simulink model "bidirection_buck_boost"  (R2025a)
settings: Solver=VariableStepAuto  StartTime=0.0  StopTime=0.1  MaxStep=1e-7  RelTol=1e-3
libraries: ee_lib x12, nesl_utility x12, fl_lib x11, spsPWMGeneratorDCDCLib x4, spsPVArrayLib x1, spspowerguiLib x1
settings Model: Creator=GNKRISHNAN  LastModifiedBy=GNKRISHNAN

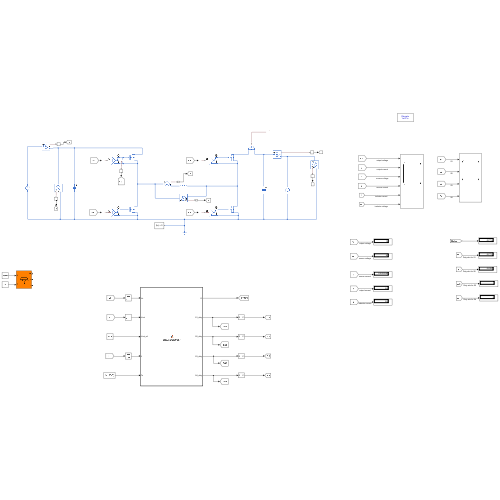
[thumbnail: Simulink's stored preview of the top-level diagram]
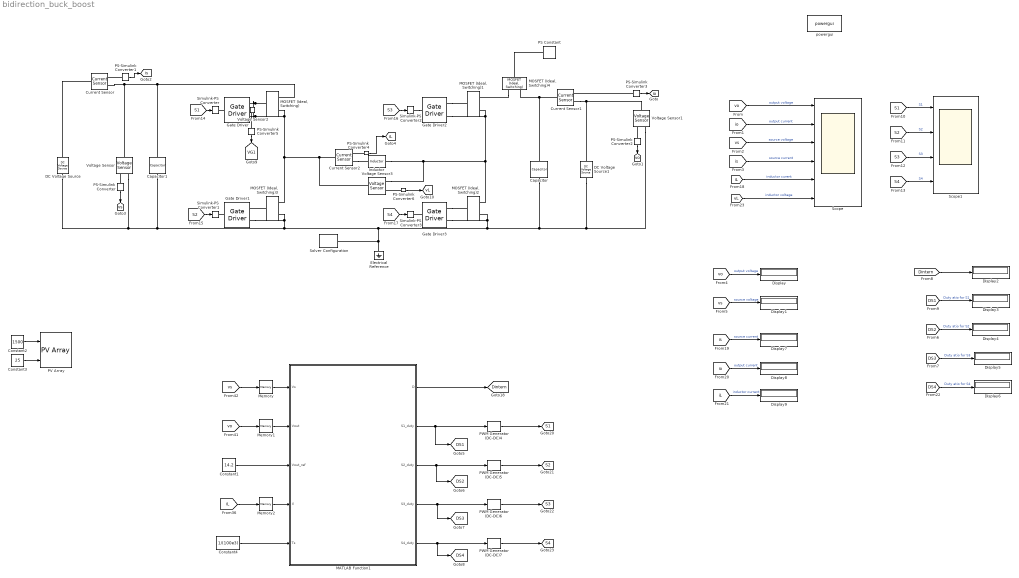
== system bidirection_buck_boost ==
  Capacitor : fl_lib/Electrical/Electrical Elements/Capacitor  c=120e-6 F  r=1e-6 Ohm  g=0 1/Ohm  i_specify=off  i_priority=None  i=0 A  i_nominal_specify=off  i_nominal_value=1  i_nominal_unit=A  v_specify=off  v_priority=None  v=0 V  v_nominal_specify=off  v_nominal_value=1  v_nominal_unit=V  vc_specify=on  vc_priority=High  vc=12 V  vc_nominal_specify=off  vc_nominal_value=1  vc_nominal_unit=V
  Capacitor1 : fl_lib/Electrical/Electrical Elements/Capacitor  c=400e-6 F  r=1e-6 Ohm  g=0 1/Ohm  i_specify=off  i_priority=None  i=0 A  i_nominal_specify=off  i_nominal_value=1  i_nominal_unit=A  v_specify=off  v_priority=None  v=0 V  v_nominal_specify=off  v_nominal_value=1  v_nominal_unit=V  vc_specify=off  vc_priority=High  vc=0 V  vc_nominal_specify=off  vc_nominal_value=1  vc_nominal_unit=V
  Constant1 : Constant  Value=14.2
  Constant2 : Constant  Value=1500
  Constant3 : Constant  Value=25
  Constant4 : Constant  Value=1/(100e3)
  Current Sensor : fl_lib/Electrical/Electrical Sensors/Current Sensor
  Current Sensor1 : fl_lib/Electrical/Electrical Sensors/Current Sensor
  Current Sensor2 : fl_lib/Electrical/Electrical Sensors/Current Sensor
  DC Voltage Source : ee_lib/Additional Components/SPICE Sources/DC Voltage Source  DC=20 V
  DC Voltage Source1 : ee_lib/Additional Components/SPICE Sources/DC Voltage Source  DC=12 V
  Display{,1..9} (10 alike) : Display
  Electrical Reference : fl_lib/Electrical/Electrical Elements/Electrical Reference
  Gate Driver{,1..3} (4 alike) : ee_lib/Semiconductors & Converters/Gate Driver  port_option=ee.enum.controlport.ps  uHigh=2.0 V  uLow=0.8 V  uHighValue=0.7  uLowValue=0.3  vHigh=15 V  vLow=0 V  tHigh=300 ns  tLow=300 ns  parameterization=ee.enum.semiconductors.gateDriverParam.outputImpedance  rHigh=2 Ohm  rLow=2 Ohm  tRise=20 ns  tFall=20 ns  cLoad=10 nF  ZonTime_specify=off  ZonTime_priority=None  ZonTime=0 s  ZoffTime_specify=off  ZoffTime_priority=None  ZoffTime=0 s
      settings: InternalSimscapePortConfiguration="{\"Bottom\":[],\"Left\":[{\"id\":\"u\",\"label\":\"u\",\"type\":\"input\"}],\"Right\":[{\"id\":\"G\",\"label\":\"G\",\"type\":\"foundation.electrical.electrical\"},{\"id\":\"S\",\"label\":\"S\",\"type\":\"foundation.electrical.electrical\"}],\"Top\":[]}"
  Inductor : ee_lib/Passive/Inductor  l=110e-6 H  enable_L_tol=ee.enum.toleranceApplication.none  L_tol=20  tol_distribution=ee.enum.toleranceDistribution.uniform  nSigma=4  r=0 Ohm  g=1e-9 1/Ohm  enable_operating_limits=ee.enum.enable.no  operating_limit_action=ee.enum.passive.reportOpLim.warn  max_working_current=1 A  power_rating=1 W  i_L_specify=off  i_L_priority=High  i_L=0 A  i_L_nominal_specify=off  i_L_nominal_value=1  i_L_nominal_unit=A
  MATLAB Function1 : MATLAB Function  TreatAsAtomicUnit=on  SystemSampleTime=1/(100e3)
  MOSFET (Ideal, Switching){,1..3} (4 alike) : ee_lib/Semiconductors & Converters/MOSFET (Ideal, Switching)  port_option=ee.enum.controlport.elec  Rds=0.01 Ohm  Goff=1e-6 1/Ohm  Vth=2 V  diode_param=ee.enum.semiconductors.protectionDiode.nodynamics  diode_Vf=0.8 V  diode_Ron=0.001 Ohm  diode_Goff=1e-5 1/Ohm  diode_C=50e-9 F  diode_iRM=-235 A  diode_iF=300 A  diode_idot=-50 A/us  diode_trr_param=ee.enum.converters.diodeReverseParam.trr_factor  diode_trr_factor=3  diode_trr=15 us  diode_Qrr=1500 s*uA  ids_specify=off  ids_priority=None  ids=0 A  ids_nominal_specify=off  ids_nominal_value=1  ids_nominal_unit=A  vds_specify=off  vds_priority=None  vds=0 V  vds_nominal_specify=off  vds_nominal_value=1  vds_nominal_unit=V  vgs_specify=off  vgs_priority=None  vgs=0 V  vgs_nominal_specify=off  vgs_nominal_value=1  vgs_nominal_unit=V  thermal_loss_option=ee.enum.converters.thermalLossOption.constantvalues  Von_data=[0, 1.8, 3.2, 6, 10, 16; 0, 2, 5.5, 9.5, 15, 25] V  Tj=[298.15, 448.15] K  Iout_data=[0, 20, 40, 60, 80, 100] A  Eon_data=[0, 55.04, 124.57, 235.53, 362.12; 0, 71.25, 161.25, 304.88, 468.75] * 1e-6 J  Eoff_data=[0, 18, 30, 56.1, 76.5; 0, 22.5, 37.5, 70.13, 95.63] * 1e-6 J  Eon_data_3D=[zeros(2, 5, 3)] J  Eoff_data_3D=[zeros(2, 5, 3)] J  Tj_loss=[298.15, 448.15] K  Iout_data_loss=[0, 10, 20, 30, 40] A  tabulateWithVds=false  Vds_loss=[0, 150, 300] V  Eon_scalar=22.86e-3 J  Eoff_scalar=17.14e-3 J  Voff=300 V  Iout_scalar=600 A  useCurrentFromPreviousCycle=false  useVoltageFromPreviousCycle=false  diodeModelType=ee.enum.converters.diodeModelType.pwl  diodeTableType=ee.enum.diode.tableType.IfMat  diode_ReverseIVType=ee.enum.diode.diodeReverseIV.constant  diode_IfMat=[.07, .12, .19, 1.75, 4.24, 7.32, 11.2; .16, .3, .72, 2.14, 4.02, 6.35, 9.12] A  diode_VfMat=[.9, 1.15, 1.25, 1.5, 1.75, 2.17, 2.6, 2.85; .58, .68, .75, 1.1, 1.38, 1.77, 2.27, 2.7] V  diode_TjVec=[25, 125] degC  diode_VfVec=[.5, .7, .9, 1.3, 1.7, 2.1, 2.5] V  diode_IfVec=[.1, .2, .5, 1, 2, 4, 7, 10] A  diode_IrMat=[1e-06, 2e-06, 5e-06, 1e-05, 2.5e-05, 5e-05, .0001; 2e-06, 5e-06, 1e-05, 4e-05, 8e-05, .0002, .0005] A  diode_VrMat=[10, 100, 200, 250, 300, 325, 350; 10, 70, 160, 220, 270, 300, 320] V  diode_VrVec=[10, 20, 40, 50, 70, 80, 100] V  diode_IrVec=[1e-06, 2e-06, 5e-06, 1e-05, 2e-05, 5e-05, .0001] A  diode_Vr=-600 V  diode_Ls=150 nH  diode_Erec=0.03 J  diode_rec_loss_model=ee.enum.diode.reverseRecoveryModel.fixed  diode_ErecVal=0 J  diode_scaleWithIandV=true  diode_ErecMat=zeros(2, 3) J  diode_TjrecVec=[298.15, 398.15] K  diode_IfrecVec=[.1, 1, 10] A  diode_IrecVal=10 A  diode_VrecVal=10 V  diode_tFilter=1 / 1000 / 100 s  separateThermalPortForDiode=false  thermal_network_parameterization=ee.enum.thermalNetworkTopology.external  Rth=[.03, .2] K/W  Rth_Cauer=[.03, .1, .2] K/W  Rth_Foster=[.08, .14, .22, .16] K/W  thermal_mass_parameterization=ee.enum.thermalNetwork.timeconstant  thermal_mass=[3, 25] J/K  thermal_mass_Cauer=[3, 10, 25] J/K  thermal_mass_Foster=[.001, .005, .05, .5] J/K  thermal_time_constant=[.1, 5] s  thermal_time_constant_Cauer=[.1, 1, 5] s  thermal_time_constant_Foster=[7e-05, .0007, .01, .08] s  thermal_mass_initial_temperatures=[25, 25] degC  thermal_mass_initial_temperatures_Cauer=[25, 25, 25] degC  junction_thermal_mass=0.1 J/K  Tvec_initial_Foster=[25, 25, 25, 25] degC  RthDiode=[.03, .2] K/W  RthCauerDiode=[.03, .1, .2] K/W  RthFosterDiode=[.03, .2] K/W  thermalMassDiode=[3, 25] J/K  thermalMassCauerDiode=[3, 10, 25] J/K  thermalMassFosterDiode=[33, 50] J/K  thermalTauDiode=[.1, 5] s  thermalTauCauerDiode=[.1, 1, 5] s  thermalTauFosterDiode=[1, 10] s  thermalMassInitTempDiode=[25, 25] degC  thermalMassInitTempCauerDiode=[25, 25, 25] degC  junctionthermalMassDiode=0.1 J/K  TVecInitialFosterDiode=[25, 25, 25, 25] degC  no_thermal_network=0  mosfet_junction_temperature_specify=off  mosfet_junction_temperature_priority=None  mosfet_junction_temperature=25 degC  mosfet_junction_temperature_nominal_specify=off  mosfet_junction_temperature_nominal_value=1  mosfet_junction_temperature_nominal_unit=degC  diode_junction_temperature_specify=off  diode_junction_temperature_priority=None  diode_junction_temperature=25 degC  diode_junction_temperature_nominal_specify=off  diode_junction_temperature_nominal_value=1  diode_junction_temperature_nominal_unit=degC  Qj_specify=off  Qj_priority=None  Qj=0 W  Qj_nominal_specify=off  Qj_nominal_value=1  Qj_nominal_unit=W  accumulatedSwitchingLosses_specify=off  accumulatedSwitchingLosses_priority=None  accumulatedSwitchingLosses=0 J
      settings: InternalSimscapePortConfiguration="{\"Bottom\":[],\"Left\":[{\"id\":\"G_elec\",\"label\":\"\",\"type\":\"foundation.electrical.electrical\"}],\"Right\":[{\"id\":\"D\",\"label\":\"\",\"type\":\"foundation.electrical.electrical\"},{\"id\":\"S\",\"label\":\"\",\"type\":\"foundation.electrical.electrical\"}],\"Top\":[]}"
  "MOSFET (Ideal, Switching)4" : ee_lib/Semiconductors & Converters/MOSFET (Ideal, Switching)  port_option=ee.enum.controlport.ps  Rds=0.01 Ohm  Goff=1e-6 1/Ohm  Vth=2 V  diode_param=ee.enum.semiconductors.protectionDiode.nodynamics  diode_Vf=0.8 V  diode_Ron=0.001 Ohm  diode_Goff=1e-5 1/Ohm  diode_C=50e-9 F  diode_iRM=-235 A  diode_iF=300 A  diode_idot=-50 A/us  diode_trr_param=ee.enum.converters.diodeReverseParam.trr_factor  diode_trr_factor=3  diode_trr=15 us  diode_Qrr=1500 s*uA  ids_specify=off  ids_priority=None  ids=0 A  ids_nominal_specify=off  ids_nominal_value=1  ids_nominal_unit=A  vds_specify=off  vds_priority=None  vds=0 V  vds_nominal_specify=off  vds_nominal_value=1  vds_nominal_unit=V  vgs_specify=off  vgs_priority=None  vgs=0 V  vgs_nominal_specify=off  vgs_nominal_value=1  vgs_nominal_unit=V  thermal_loss_option=ee.enum.converters.thermalLossOption.constantvalues  Von_data=[0, 1.8, 3.2, 6, 10, 16; 0, 2, 5.5, 9.5, 15, 25] V  Tj=[298.15, 448.15] K  Iout_data=[0, 20, 40, 60, 80, 100] A  Eon_data=[0, 55.04, 124.57, 235.53, 362.12; 0, 71.25, 161.25, 304.88, 468.75] * 1e-6 J  Eoff_data=[0, 18, 30, 56.1, 76.5; 0, 22.5, 37.5, 70.13, 95.63] * 1e-6 J  Eon_data_3D=[zeros(2, 5, 3)] J  Eoff_data_3D=[zeros(2, 5, 3)] J  Tj_loss=[298.15, 448.15] K  Iout_data_loss=[0, 10, 20, 30, 40] A  tabulateWithVds=false  Vds_loss=[0, 150, 300] V  Eon_scalar=22.86e-3 J  Eoff_scalar=17.14e-3 J  Voff=300 V  Iout_scalar=600 A  useCurrentFromPreviousCycle=false  useVoltageFromPreviousCycle=false  diodeModelType=ee.enum.converters.diodeModelType.pwl  diodeTableType=ee.enum.diode.tableType.IfMat  diode_ReverseIVType=ee.enum.diode.diodeReverseIV.constant  diode_IfMat=[.07, .12, .19, 1.75, 4.24, 7.32, 11.2; .16, .3, .72, 2.14, 4.02, 6.35, 9.12] A  diode_VfMat=[.9, 1.15, 1.25, 1.5, 1.75, 2.17, 2.6, 2.85; .58, .68, .75, 1.1, 1.38, 1.77, 2.27, 2.7] V  diode_TjVec=[25, 125] degC  diode_VfVec=[.5, .7, .9, 1.3, 1.7, 2.1, 2.5] V  diode_IfVec=[.1, .2, .5, 1, 2, 4, 7, 10] A  diode_IrMat=[1e-06, 2e-06, 5e-06, 1e-05, 2.5e-05, 5e-05, .0001; 2e-06, 5e-06, 1e-05, 4e-05, 8e-05, .0002, .0005] A  diode_VrMat=[10, 100, 200, 250, 300, 325, 350; 10, 70, 160, 220, 270, 300, 320] V  diode_VrVec=[10, 20, 40, 50, 70, 80, 100] V  diode_IrVec=[1e-06, 2e-06, 5e-06, 1e-05, 2e-05, 5e-05, .0001] A  diode_Vr=-600 V  diode_Ls=150 nH  diode_Erec=0.03 J  diode_rec_loss_model=ee.enum.diode.reverseRecoveryModel.fixed  diode_ErecVal=0 J  diode_scaleWithIandV=true  diode_ErecMat=zeros(2, 3) J  diode_TjrecVec=[298.15, 398.15] K  diode_IfrecVec=[.1, 1, 10] A  diode_IrecVal=10 A  diode_VrecVal=10 V  diode_tFilter=1 / 1000 / 100 s  separateThermalPortForDiode=false  thermal_network_parameterization=ee.enum.thermalNetworkTopology.external  Rth=[.03, .2] K/W  Rth_Cauer=[.03, .1, .2] K/W  Rth_Foster=[.08, .14, .22, .16] K/W  thermal_mass_parameterization=ee.enum.thermalNetwork.timeconstant  thermal_mass=[3, 25] J/K  thermal_mass_Cauer=[3, 10, 25] J/K  thermal_mass_Foster=[.001, .005, .05, .5] J/K  thermal_time_constant=[.1, 5] s  thermal_time_constant_Cauer=[.1, 1, 5] s  thermal_time_constant_Foster=[7e-05, .0007, .01, .08] s  thermal_mass_initial_temperatures=[25, 25] degC  thermal_mass_initial_temperatures_Cauer=[25, 25, 25] degC  junction_thermal_mass=0.1 J/K  Tvec_initial_Foster=[25, 25, 25, 25] degC  RthDiode=[.03, .2] K/W  RthCauerDiode=[.03, .1, .2] K/W  RthFosterDiode=[.03, .2] K/W  thermalMassDiode=[3, 25] J/K  thermalMassCauerDiode=[3, 10, 25] J/K  thermalMassFosterDiode=[33, 50] J/K  thermalTauDiode=[.1, 5] s  thermalTauCauerDiode=[.1, 1, 5] s  thermalTauFosterDiode=[1, 10] s  thermalMassInitTempDiode=[25, 25] degC  thermalMassInitTempCauerDiode=[25, 25, 25] degC  junctionthermalMassDiode=0.1 J/K  TVecInitialFosterDiode=[25, 25, 25, 25] degC  no_thermal_network=0  mosfet_junction_temperature_specify=off  mosfet_junction_temperature_priority=None  mosfet_junction_temperature=25 degC  mosfet_junction_temperature_nominal_specify=off  mosfet_junction_temperature_nominal_value=1  mosfet_junction_temperature_nominal_unit=degC  diode_junction_temperature_specify=off  diode_junction_temperature_priority=None  diode_junction_temperature=25 degC  diode_junction_temperature_nominal_specify=off  diode_junction_temperature_nominal_value=1  diode_junction_temperature_nominal_unit=degC  Qj_specify=off  Qj_priority=None  Qj=0 W  Qj_nominal_specify=off  Qj_nominal_value=1  Qj_nominal_unit=W  accumulatedSwitchingLosses_specify=off  accumulatedSwitchingLosses_priority=None  accumulatedSwitchingLosses=0 J
  Memory : Memory
  Memory1 : Memory
  Memory2 : Memory
  PS Constant : fl_lib/Physical Signals/Sources/PS Constant  constant=0 V
  PS-Simulink Converter{,1..6} (7 alike) : nesl_utility/PS-Simulink Converter  PhysicalDomain=network_engine_domain  SubClassName=ps_output  LeftPortType=input  RightPortType=output  PseudoPeriodic=off  Frequencies=[]  VectorFormat=inherit  Unit=inherit  AffineConversion=off
  PV Array : spsPVArrayLib/PV Array  Npar=1  Nser=1  PlotType=one module @ 25 deg.C & specified irradiances  S_vec="[ 1000  500  100 ]"  Temp_C_vec="[ 45 25  ]"  ModuleName=User-defined  PlotWhenSelected=off  Pm=130.032  Ncell=60  Voc=21.6  Isc=8.36  Vm=17.2  Im=7.56  beta_Voc_pc=-0.1  alpha_Isc_pc=0.001  beta_Voc=-0.0216  alpha_Isc=8.36e-05  IL=8.428  I0=1.3766e-16  nI=0.36322  Rsh=37.2573  Rs=0.33372  RobustModel=off  RobustCellTemperature=313.3991  BAL=on  Tc=1e-6  Tfilter=5e-5
  PWM Generator (DC-DC){4..7} (4 alike) : spsPWMGeneratorDCDCLib/PWM Generator (DC-DC)  Fsw=100e3  Ts=0
  Scope : Scope  NumInputPorts=6
      settings: ActiveDisplayYMinimum=2  ActiveDisplayYMaximum=22
  Scope1 : Scope  NumInputPorts=4
      settings: ActiveDisplayYMinimum=-0.12499999999999997  ActiveDisplayYMaximum=1.125
  Simulink-PS Converter{,1..3} (4 alike) : nesl_utility/Simulink-PS Converter  PhysicalDomain=network_engine_domain  SubClassName=ps_input  LeftPortType=input  RightPortType=output  PseudoPeriodic=off  Frequencies=[]  NoiseDistribution=none  NoiseParameters=[]  Unit=1  AffineConversion=off  FilteringAndDerivatives=provide  SimscapeFilterOrder=1  InputFilterTimeConstant=0.001  UdotUserProvided=0
  Solver Configuration : nesl_utility/Solver Configuration  PhysicalDomain=network_engine_domain  SubClassName=solver  LeftPortType=input  RightPortType=generic  Tones=[]  Harmonics=[]  SimulateNoise=off  Profile=off  UseLocalSampling=off  EnableSwitchedLinearOptims=on  FrequencyDomain=off  UseCCode=off  RelTol=0.001  AbsTol=0.001  MinStep=1e-09  ToWorkspace=off  RevertToSquareIcSolve=off  NumHomotopyIterations=100  PhasorMode=off  PhasorModeNumHarmonics=1  ConsistencySolver=NEWTON_XTOL_AFTER_FTOL  IndexReductionMethod=DerivativeReplacement  DoDC=off  ResidualTolerance=1e-09  ConsistencyTolSource=GLOBAL  ConsistencyAbsTol=0.001  ConsistencyRelTol=0.001  ConsistencyTolFactor=0.001  UseLocalSolver=off  LocalSolverChoice=NE_BACKWARD_EULER_ADVANCER  ResolveIndetEquations=on  FunctionEvalNumThread=1  LocalSolverSampleTime=0.001  DoFixedCost=off  MaxNonlinIter=3  MaxModeIter=2  ComputeImpulses=off  ImpulseIterations=2  LinearAlgebra=auto  LinearAlgebraNumThread=0  EquationFormulation=NE_TIME_EF  DelaysMemoryBudget=1024  AutomaticFiltering=on  FilteringTimeConstant=0.001  PartitionStorageMethod=AS_NEEDED  PartitionMemoryBudget=1024  PartitionMethod=ROBUST  MultibodyUseLocalSolver=off  MultibodyLocalSolverChoice=ODE1  MultibodyLocalSolverSampleTime=0.001
  Voltage Sensor{,1..3} (4 alike) : fl_lib/Electrical/Electrical Sensors/Voltage Sensor
  powergui : spspowerguiLib/powergui  Priority=1  SimulationMode=Discrete  SampleTime=1e-7  frequency=60  Iterations=50  frequencyindice=60  Pbase=100e6  ErrMax=1e-4  UnitsV=kV  UnitsW=MW  buscounter=0  FunctionMessages=off  echomessages=off  EnableUseOfTLC=off  CurrentSourceSwitches=off  DisableSnubberDevices=off  DisableRonSwitches=off  DisableVfSwitches=off  DisplayEquations=off  AutomaticDiscreteSolvers=off  SolverType=Tustin/Backward Euler (TBE)  Interpol=off  ExternalGateDelay=off  methode=off  Ts=100  x0status=blocks  SPID=on  SwTol=0  HookPort=off  NonlinearTolerance=1e-4  nMaxIteration=100  ContinueOnMaxIteration=off  RestoreLinks=warning  ResistiveCurrentMeasurement=off  Frange=[0:2:500]  Ylog=off  Xlog=on  ShowGrid=off  save=off  variable=ZData  structure=0  ZoomFFT=off  StartTime=0.0  cycles=1  DisplayStyle=1  fundamental=60  FreqAxis=off  MaxFrequency=1000  frequencyindicesteady=1  RmsSteady=1  display=off
  tag scope: DS1=global, DS2=global, DS3=global, DS4=global, Dintern=global, S1=global, S2=global, S3=global, S4=global, VG1=global, iL=global, io=global, is=global, vL=global, vo=global, vs=global
  wires:
  [DS2] -> Display4/1  "Duty atio for S2"
  [DS4] -> Display6/1  "Duty atio for S4"
  [S2] -> Scope1/2  "S2"
  Memory/1 -> MATLAB Function1/1(Vs)
  Constant1/1 -> MATLAB Function1/3(Vout_ref)
  [Dintern] -> Display2/1
  [vs] -> Scope/3  "source voltage"
  MATLAB Function1/1(D) -> [Dintern]
  PWM Generator (DC-DC)7/1 -> [S4]
  Memory1/1 -> MATLAB Function1/2(Vout)
  [vo] -> Memory1/1
  [S1] -> Simulink-PS Converter/1
  [S4] -> Scope1/4  "S4"
  [S3] -> Simulink-PS Converter2/1
  Constant4/1 -> MATLAB Function1/5(Ts)
  PS-Simulink Converter2/1 -> [vo]
  [iL] -> Scope/5  "inductor curent"
  MATLAB Function1/3(S2_duty) -> [DS2], PWM Generator (DC-DC)5/1
  PWM Generator (DC-DC)4/1 -> [S1]
  PS-Simulink Converter1/1 -> [is]
  [vs] -> Memory/1
  [S1] -> Scope1/1  "S1"
  Memory2/1 -> MATLAB Function1/4(Il)
  [io] -> Scope/2  "output current"
  PS-Simulink Converter4/1 -> [iL]
  MATLAB Function1/5(S4_duty) -> [DS4], PWM Generator (DC-DC)7/1
  [S3] -> Scope1/3  "S3"
  MATLAB Function1/2(S1_duty) -> [DS1], PWM Generator (DC-DC)4/1
  MATLAB Function1/4(S3_duty) -> [DS3], PWM Generator (DC-DC)6/1
  [DS1] -> Display3/1  "Duty atio for S1"
  [iL] -> Memory2/1
  [is] -> Scope/4  "source current"
  [vo] -> Display/1  "output voltage"
  PWM Generator (DC-DC)6/1 -> [S3]
  PWM Generator (DC-DC)5/1 -> [S2]
  [S4] -> Simulink-PS Converter3/1
  PS-Simulink Converter/1 -> [vs]
  PS-Simulink Converter3/1 -> [io]
  [DS3] -> Display5/1  "Duty atio for S3"
  [vs] -> Display1/1  "source voltage"
  [S2] -> Simulink-PS Converter1/1
  [vo] -> Scope/1  "output voltage"
  [io] -> Display8/1  "output current"
  [is] -> Display7/1  "source current"
  [iL] -> Display9/1  "inductor current"
  PS-Simulink Converter5/1 -> [VG1]
  PS-Simulink Converter6/1 -> [vL]
  [vL] -> Scope/6  "inductor voltage"
  Constant3/1 -> PV Array/2
  Constant2/1 -> PV Array/1
  connections:
  Electrical Reference/LConn1 -- Capacitor1/RConn1 -- Voltage Sensor/RConn2 -- DC Voltage Source/RConn1 -- "MOSFET (Ideal, Switching)3"/RConn2 -- Gate Driver1/RConn2 -- "MOSFET (Ideal, Switching)2"/RConn2 -- Gate Driver3/RConn2 -- DC Voltage Source1/RConn1 -- Voltage Sensor1/RConn2 -- Capacitor/RConn1 -- Solver Configuration/RConn1
  "MOSFET (Ideal, Switching)"/RConn1 -- Voltage Sensor/LConn1 -- Current Sensor/RConn2 -- Capacitor1/LConn1
  DC Voltage Source1/LConn1 -- Current Sensor1/RConn2 -- Voltage Sensor1/LConn1
  Capacitor/LConn1 -- Current Sensor1/LConn1 -- "MOSFET (Ideal, Switching)4"/RConn1
  "MOSFET (Ideal, Switching)2"/RConn1 -- Voltage Sensor3/RConn2 -- Inductor/RConn1 -- "MOSFET (Ideal, Switching)1"/RConn2 -- Gate Driver2/RConn2
  "MOSFET (Ideal, Switching)"/RConn2 -- Voltage Sensor2/RConn2 -- Gate Driver/RConn2 -- Voltage Sensor3/LConn1 -- Current Sensor2/LConn1 -- "MOSFET (Ideal, Switching)3"/RConn1
  DC Voltage Source/LConn1 -- Current Sensor/LConn1
  PS-Simulink Converter4/LConn1 -- Current Sensor2/RConn1
  "MOSFET (Ideal, Switching)3"/LConn1 -- Gate Driver1/RConn1
  Gate Driver2/RConn1 -- "MOSFET (Ideal, Switching)1"/LConn1
  "MOSFET (Ideal, Switching)4"/RConn2 -- "MOSFET (Ideal, Switching)1"/RConn1
  Current Sensor2/RConn2 -- Inductor/LConn1
  Gate Driver3/RConn1 -- "MOSFET (Ideal, Switching)2"/LConn1
  PS-Simulink Converter3/LConn1 -- Current Sensor1/RConn1
  PS Constant/RConn1 -- "MOSFET (Ideal, Switching)4"/LConn1
  Simulink-PS Converter1/RConn1 -- Gate Driver1/LConn1
  Gate Driver3/LConn1 -- Simulink-PS Converter3/RConn1
  PS-Simulink Converter1/LConn1 -- Current Sensor/RConn1
  Gate Driver/LConn1 -- Simulink-PS Converter/RConn1
  Simulink-PS Converter2/RConn1 -- Gate Driver2/LConn1
  PS-Simulink Converter2/LConn1 -- Voltage Sensor1/RConn1
  "MOSFET (Ideal, Switching)"/LConn1 -- Voltage Sensor2/LConn1 -- Gate Driver/RConn1
  PS-Simulink Converter/LConn1 -- Voltage Sensor/RConn1
  Voltage Sensor2/RConn1 -- PS-Simulink Converter5/LConn1
  PS-Simulink Converter6/LConn1 -- Voltage Sensor3/RConn1

== matlab function bidirection_buck_boost/MATLAB Function1 ==
  data: Vs input; D output; S1_duty output; S2_duty output; Vout input; Vout_ref input; Il input; S3_duty output; S4_duty output; Ts input
function [D, S1_duty, S2_duty, S3_duty, S4_duty] = biDirBuckController(Vs, Vout, Vout_ref, Il, Ts)
% Codegen-safe digital controller for 4-switch bidirectional DC-DC (buck only with hysteresis buck-boost)

% -------- Persistent Parameters --------
persistent Kp_v Ki_v Kp_i Ki_i Dmax Il_max hyst ...
           v_int i_int Iref_min Iref_max

if isempty(Kp_v)
    % PI Gains
    Kp_v = 0.8;   Ki_v = 120;   % Voltage loop gains
    Kp_i = 0.03;  Ki_i = 300;   % Current loop gains
    
    % Limits
    Dmax     = 0.98;   % duty saturation
    Il_max   = 8.5;    % A, current limit
    hyst     = 0.5;    % hysteresis band in volts
    Iref_min = 0.0;    % min ref current
    Iref_max = Il_max; % max ref current
    
    % States
    v_int = 0.0;   % voltage PI integrator
    i_int = 0.0;   % current PI integrator
end

% -------- Output defaults (safe) --------
D       = 0.0;
S1_duty = 0.0;
S2_duty = 0.0;
S3_duty = 0.0;
S4_duty = 0.0;

% -------- Determine Region --------
if Vs > (Vout + hyst)
    region = 1; % Buck
elseif abs(Vs - Vout) <= hyst
    region = 2; % Buck-Boost
else
    region = 0; % Idle
end

% -------- Outer Voltage Loop --------
v_err = Vout_ref - Vout;
v_int = v_int + Ki_v * v_err * Ts;  % integrator update
Iref  = v_int + Kp_v * v_err;       % PI output

% Clamp Iref
if Iref > Iref_max, Iref = Iref_max; end
if Iref < Iref_min, Iref = Iref_min; end

% Hard limit: if Il > Il_max, reduce reference
if Il >= Il_max
    Iref = min(Iref, Il_max);
end

% -------- Inner Current Loop --------
i_err = Iref - Il;
i_int = i_int + Ki_i * i_err * Ts;
u_p   = Kp_i * i_err;

duty_raw = i_int + u_p;

% Saturation and anti-windup
if duty_raw > Dmax
    D     = Dmax;
    i_int = D - u_p;
elseif duty_raw < 0
    D     = 0.0;
    i_int = -u_p;
else
    D     = duty_raw;
end

% -------- Duty Mapping --------
switch region
    case 1 % Buck
        S1_duty = D;
        S2_duty = 1 - D;
        S3_duty = 1.0;
        S4_duty = 0.0;
    case 2 % Buck-Boost
        S1_duty = D;
        S4_duty = D;
        S2_duty = 1 - D;
        S3_duty = 1 - D;
    otherwise % Idle
        S1_duty = 0.0;
        S2_duty = 0.0;
        S3_duty = 0.0;
        S4_duty = 0.0;
end

% Clamp (safety)
if S1_duty > 1, S1_duty = 1; elseif S1_duty < 0, S1_duty = 0; end
if S2_duty > 1, S2_duty = 1; elseif S2_duty < 0, S2_duty = 0; end
if S3_duty > 1, S3_duty = 1; elseif S3_duty < 0, S3_duty = 0; end
if S4_duty > 1, S4_duty = 1; elseif S4_duty < 0, S4_duty = 0; end

% -------- Store back states --------
% (codegen supports reassigning persistent scalars)
% all updated states written back
end
